simulink model "quadcopter_model"  (Simulink 8.6)
settings: Solver=VariableStepAuto  StartTime=0.0  StopTime=2  RelTol=1e-3
values from neighbouring files (symbols this model uses):
  A = [0.25 ... (first row only)    [quadcopter_init.m]
  b = 1.140e-7    (= 1.14e-07)    [linearization.m]    (also in quadcopter_init.m)
  g = 9.81    [linearization.m]    (also in quadcopter_init.m)
  I = [4.856e-3 ... (first row only)    [quadcopter_init.m]
  k = 2.980e-6    (= 2.98e-06)    [linearization.m]    (also in quadcopter_init.m)
  l = 0.225    [linearization.m]    (also in quadcopter_init.m)
  m = 0.468    [linearization.m]    (also in quadcopter_init.m)
settings Model: Creator=Daniel  LastModifiedBy=mgreiff
settings DataIOCC: SaveFormat=Dataset  SignalLoggingSaveFormat=Dataset
settings OptimizationCC: ExpressionDepthLimit=128
settings DebuggingCC: UnderspecifiedInitializationDetection=Simplified  MergeDetectMultiDrivingBlocksExec=error  SolverPrmCheckMsg=none  FcnCallInpInsideContextMsg=EnableAllAsError  StateNameClashWarn=none
settings HardwareCC: ProdBitPerPointer=64  ProdLargestAtomicFloat=Float  ProdIntDivRoundTo=Zero  ProdEndianess=LittleEndian  ProdWordSize=64  ProdHWDeviceType=Intel->x86-64 (Windows64)
settings GRTTargetCC: GeneratePreprocessorConditionals=Use local settings  CombineOutputUpdateFcns=on  GRTInterface=off
settings ConfigComp: CovModelRefEnable=off

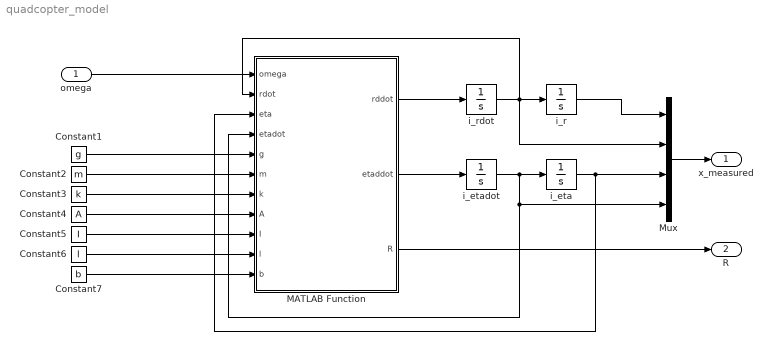
== system quadcopter_model ==
  omega : Inport  PortDimensions=4
  Constant1 : Constant  Value=g
  Constant2 : Constant  Value=m
  Constant3 : Constant  Value=k
  Constant4 : Constant  Value=A
  Constant5 : Constant  Value=I
  Constant6 : Constant  Value=l
  Constant7 : Constant  Value=b
  MATLAB Function : MATLAB Function  TreatAsAtomicUnit=on
  Mux : Mux
  i_eta : Integrator  InitialCondition=[0 0 0]'
  i_etadot : Integrator  InitialCondition=[0; 0; 0]
  i_r : Integrator  InitialCondition=[0 0 0]'
  i_rdot : Integrator  InitialCondition=[0; 0; 0]
  x_measured : Outport
  R : Outport  Port=2
  wires:
  MATLAB Function/2(etaddot) -> i_etadot/1
  MATLAB Function/1(rddot) -> i_rdot/1
  i_rdot/1 -> Mux/2, MATLAB Function/2(rdot), i_r/1
  i_etadot/1 -> MATLAB Function/4(etadot), Mux/4, i_eta/1
  i_eta/1 -> MATLAB Function/3(eta), Mux/3
  i_r/1 -> Mux/1
  Constant4/1 -> MATLAB Function/8(A)
  Constant3/1 -> MATLAB Function/7(k)
  Constant2/1 -> MATLAB Function/6(m)
  Constant1/1 -> MATLAB Function/5(g)
  Constant7/1 -> MATLAB Function/11(b)
  Constant6/1 -> MATLAB Function/10(l)
  Constant5/1 -> MATLAB Function/9(I)
  MATLAB Function/3(R) -> R/1
  omega/1 -> MATLAB Function/1(omega)
  Mux/1 -> x_measured/1

== matlab function MATLAB Function ==
  data: omega input double; rddot output double; rdot input double; eta input double; etadot input double; etaddot output double; g input double; m input double; k input double; A input double; I input double; l input double; b input double; R output double
function [ rddot,etaddot,R] = quad_acceleration(omega, rdot, eta, etadot, g, m, k, A, I, l, b)
    % Equations from Teppo Luukkonen, Modelling and control of quadcopter
    phi = eta(1); theta = eta(2); psi = eta(3); % Roll, pitch, yaw
    phidot = etadot(1); thetadot = etadot(2); psidot = etadot(3); % Roll, pitch, yaw
    
    T = k * sum(omega.^2); % (7)
    
    % Gravity acceleration
    Ga = -g * [0; 0; 1];
    
    % Thrust acceleration
    angM = [cos(psi)*sin(theta)*cos(phi) + sin(psi)*sin(phi);
          sin(psi)*sin(theta)*cos(phi) - cos(psi)*sin(phi);
          cos(theta)*cos(phi)];
    Ta = T/m * angM;
    
    % Drag
    Aa = -1/m * diag(A) * rdot;
    
    rddot = Ga + Ta + Aa; % (21)
    %disp([Ta rddot]);
    
    % Define the C-matrix as (19)
    Ixx = I(1); Iyy = I(2); Izz = I(3);
    Sphi = sin(phi); Stheta = sin(theta); Spsi = sin(psi);
    Cphi = cos(phi); Ctheta = cos(theta); Cpsi = cos(psi);
    
    C11 = 0;
    C12 = (Iyy - Izz) * (thetadot*Cphi*Sphi + psidot*Sphi^2*Ctheta) + (Izz - Iyy)*psidot*Cphi^2*Ctheta - Ixx*psidot*Ctheta;
    C13 = (Izz - Iyy) * psidot*Cphi*Sphi*Ctheta^2;
    C21 = (Izz - Iyy) * (thetadot*Cphi*Sphi + psidot*Sphi*Ctheta) + (Iyy - Izz)*psidot*Cphi^2*Ctheta - Ixx*psidot*Ctheta;
    C22 = (Izz - Iyy) * phidot*Cphi*Sphi;
    C23 = -Ixx * psidot * Stheta * Ctheta + Iyy * psidot * Sphi^2 * Stheta * Ctheta + Izz * psidot * Cphi^2 * Stheta * Ctheta;
    C31 = (Iyy - Izz) * psidot * Ctheta^2 * Sphi * Cphi - Ixx * thetadot * Ctheta;
    C32 = (Izz - Iyy) * (thetadot * Cphi * Sphi * Stheta + phidot * Sphi^2 * Ctheta) + (Iyy - Izz) * phidot * Cphi^2 * Ctheta...
            + Ixx * psidot * Stheta * Ctheta - Iyy * psidot * Sphi^2 * Stheta * Ctheta - Izz * psi * Cphi^2 * Stheta * Ctheta;
    C33 = (Iyy - Izz) * phidot * Cphi * Sphi * Ctheta^2 - Iyy * thetadot * Sphi^2 * Ctheta * Stheta ...
            - Izz * thetadot * Cphi^2 * Ctheta * Stheta + Ixx * thetadot * Ctheta * Stheta;
    
    C = [C11 C12 C13; C21 C22 C23; C31 C32 C33];   
    
    % (8)
    tau_phi =  l * k * (-omega(2)^2 + omega(4)^2);
    tau_theta =  l * k * (-omega(1)^2 + omega(3)^2);
    tau_psi =  -b * sum(omega(1)^2 - omega(2)^2 + omega(3)^2 - omega(4)^2); % Modified from the text, rotor 2 and 4 spin in oposite direction
    tau_b = [tau_phi; tau_theta; tau_psi];
    
    % (16)
    J11 = Ixx; J12 = 0; J13 = -Ixx*Stheta;
    J21 = 0;
    J22 = Iyy * Cphi^2 + Izz * Sphi^2;
    J23 = (Iyy - Izz) * Cphi * Sphi * Ctheta;
    J31 = -Ixx * Stheta;
    J32 = (Iyy - Izz)*Cphi*Sphi*Ctheta;
    J33 = Ixx * Stheta^2 + Iyy * Sphi^2 * Ctheta^2 + Izz * Cphi^2*Ctheta^2;
    J = [J11 J12 J13; J21 J22 J23; J31 J32 J33];  
            
    etaddot = J\(tau_b - C*etadot); % (20)
    
    R = [Cpsi*Ctheta, Cpsi*Stheta*Sphi-Spsi*Cphi, Cpsi*Stheta*Cphi + Spsi*Sphi;
        Spsi*Ctheta, Spsi*Stheta*Sphi+Cpsi*Cphi, Spsi*Stheta*Cphi - Cpsi*Sphi;
        -Stheta, Ctheta*Sphi, Ctheta*Cphi];
end
